simulink model "Parallel3"  (Simulink 8.7)
settings: Solver=ode45  StartTime=0.0  StopTime=10.0  RelTol=1e-3
settings Model: Creator=scaife  LastModifiedBy=bourbouh  ExtModeAutoUpdateStatusClock=off
settings DataIOCC: SignalLoggingSaveFormat=ModelDataLogs  SignalLoggingName=sigsOut
settings DebuggingCC: SaveWithParameterizedLinksMsg=none  SignalResolutionControl=TryResolveAllWithWarning  MultiTaskDSMMsg=warning  MultiTaskCondExecSysMsg=none
settings HardwareCC: TargetUnknown=on
settings SFSimCC: SimParseCustomCode=off
settings GRTTargetCC: GeneratePreprocessorConditionals=Use local settings  CombineOutputUpdateFcns=off  GRTInterface=on

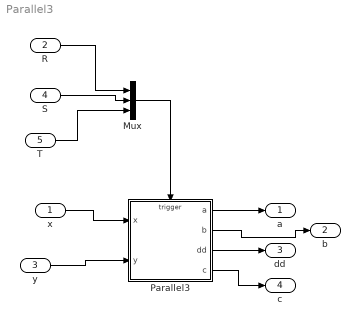
== system Parallel3 ==
  x : Inport
  R : Inport  Port=2
  y : Inport  Port=3
  S : Inport  Port=4
  T : Inport  Port=5
  Mux : Mux  Inputs=3
  Parallel3 : Stateflow chart  TreatAsAtomicUnit=on
  a : Outport
  b : Outport  Port=2
  dd : Outport  Port=3
  c : Outport  Port=4
  wires:
  Mux/1 -> Parallel3/Trigger
  T/1 -> Mux/3
  S/1 -> Mux/2
  R/1 -> Mux/1
  x/1 -> Parallel3/1(x)
  y/1 -> Parallel3/2(y)
  Parallel3/1(a) -> a/1
  Parallel3/2(b) -> b/1
  Parallel3/3(dd) -> dd/1
  Parallel3/4(c) -> c/1

== stateflow chart Parallel3 ==
  state A [parallel]
    settings: executionOrder=1
    state A1
      state A1a/
        en:a=x+1
      state A1b/
        en:a=x+2
      (default) -> A1a
      A1b -> A1a : R
      A1a -> A1b : S
    state A2
      state A2a/
        en:a=x+3
      state A2b/
        en:a=x+4
      (default) -> A2a
      A2b -> A2a : R
      A2a -> A2b : S
    (default) -> A1
    A1 -> A2 : T
    A2 -> A1 : T
  state B [parallel]
    settings: executionOrder=2
    state B2
      state B2a/
        en:b=x+7
      state B2b/
        en:b=x+8
      (default) -> B2a
      B2b -> B2a : R
      B2a -> B2b : S
    state B1
      state B1a/
        en:b=x+5
      state B1b/
        en:b=x+6
      (default) -> B1a
      B1b -> B1a : R
      B1a -> B1b : S
    (default) -> B1
    B1 -> B2 : T
    B2 -> B1 : T
  state C [parallel]
    settings: executionOrder=3
    state C2
      state C2a/
        en:c=y+3
      state C2b/
        en:c=y+4
      (default) -> C2a
      C2a -> C2b : S
      C2b -> C2a : R
    state C1
      state C1a/
        en:c=y+1
      state C1b/
        en:c=y+2
      (default) -> C1a
      C1a -> C1b : S
      C1b -> C1a : R
    (default) -> C1
    C1 -> C2 : T
    C2 -> C1 : T
  state D [parallel]
    settings: executionOrder=4
    state D2
      state D2a/
        en:dd=y+7
      state D2b/
        en:dd=y+8
      (default) -> D2a
      D2a -> D2b : S
      D2b -> D2a : R
    state D1
      state D1a/
        en:dd=y+5
      state D1b/
        en:dd=y+6
      (default) -> D1a
      D1a -> D1b : S
      D1b -> D1a : R
    (default) -> D1
    D1 -> D2 : T
    D2 -> D1 : T
  data: a output int32; b output int32; dd output int32; c output int32; x input int32; y input int32
  events: R input EITHER_EDGE_EVENT; S input EITHER_EDGE_EVENT; T input EITHER_EDGE_EVENT
